simulink model "IEEE14_bus_system_2"  (R2024a)
settings: Solver=VariableStepAuto  StartTime=0.0  StopTime=0.2  RelTol=1e-3
libraries: spsThreePhaseSeriesRLCBranchLib x120, spsThreePhaseVIMeasurementLib x51, spsGroundLib x40, spsLoadFlowBusLib x33, spsThreePhaseSeriesRLCLoadLib x24, spsThreePhaseSourceLib x10, spsThreePhaseTransformerTwoWindingsLib x5, spspowerguiLib x2
(part 1 of 3)
settings Model: Creator=SIMPATY SOLUTIONS  LastModifiedBy=Nani
settings SolverCC: AlgebraicLoopSolver=TrustRegion
settings DebuggingCC: UnconnectedInputMsg=warning  UnconnectedOutputMsg=warning  UnconnectedLineMsg=warning
settings ModelReferenceCC: EnableRefExpFcnMdlSchedulingChecks=on
settings RTWCC: GPUComputeCapability=3.5

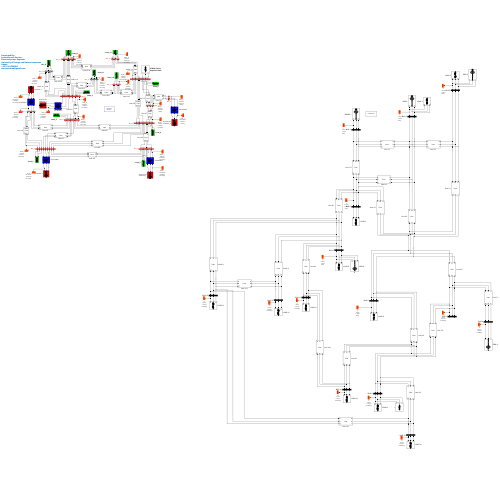
[thumbnail: Simulink's stored preview of the top-level diagram]
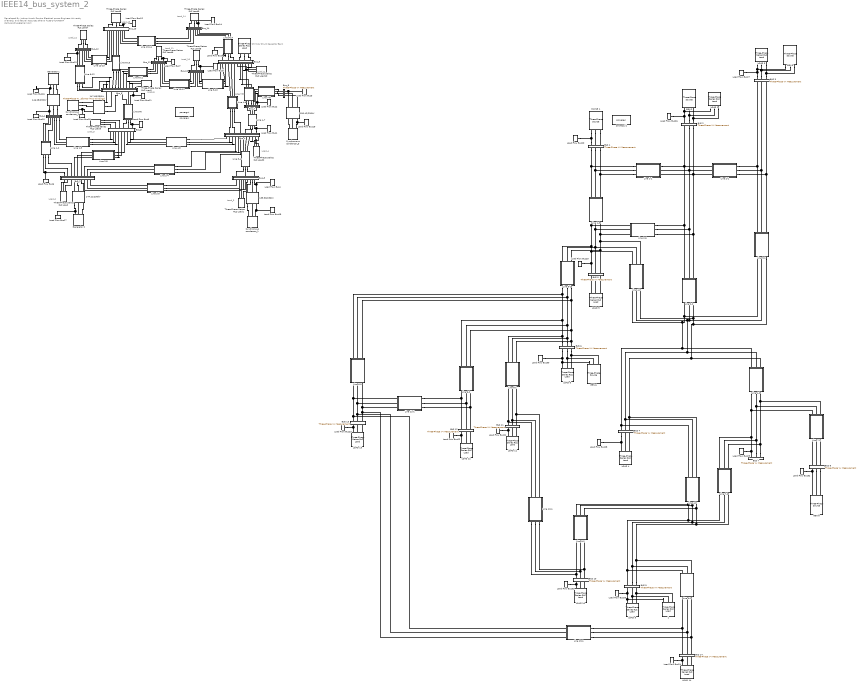
== system IEEE14_bus_system_2 ==
  note: Developed By:
      | Joshua Armah Dantuo
      | Electrical power Engineer
      | University of Energy and Natural resources
      | Ghana
      | +233-241790004
      | dantuojoshua@gmail.com
  note: 25 MVar Shunt
      | Capacitor Bank
  note: Load_4
  note: Load_3
  note: Load_5
  note: Load_9
  note: Load_11
  note: Load_10
  note: Load_12
  note: Load_6
  note: Load_13
  note: Load_14
  note: Load_2
  " " : spsThreePhaseSeriesRLCLoadLib/Three-Phase Series RLC Load  LConnTagsString=A|B|C  Configuration=Y (grounded)  NominalVoltage=230e3  Vabc=[1e3 1e3 1e3]  Vabcp=[1e3 1e3 1e3]  NominalFrequency=60  UnbalancedPower=off  ActivePower=0  InductivePower=0  CapacitivePower=25e6  Pabc=[10e3 9e3 11e3]  QLabc=[100 90 110]  QCabc=[100 90 110]  Pabcp=[10e3 9e3 11e3]  QLabcp=[100 90 110]  QCabcp=[100 90 110]  Measurements=None  LoadType=constant Z
  " 1" : spsThreePhaseSeriesRLCLoadLib/Three-Phase Series RLC Load  LConnTagsString=A|B|C  Configuration=Y (grounded)  NominalVoltage=230e3  Vabc=[1e3 1e3 1e3]  Vabcp=[1e3 1e3 1e3]  NominalFrequency=60  UnbalancedPower=off  ActivePower=0  InductivePower=0  CapacitivePower=25e6  Pabc=[10e3 9e3 11e3]  QLabc=[100 90 110]  QCabc=[100 90 110]  Pabcp=[10e3 9e3 11e3]  QLabcp=[100 90 110]  QCabcp=[100 90 110]  Measurements=None  LoadType=constant Z
  139.38/230kV : spsThreePhaseTransformerTwoWindingsLib/Three-Phase Transformer (Two Windings)  Winding1Connection=Yg  Winding2Connection=Yg  CoreType=Three single-phase transformers  SetSaturation=off  Hysteresis=off  DataFile='hysteresis'  SetInitialFlux=off  Measurements=None  UNITS=pu  NominalPower=[ 120e6 , 60 ]  Winding1=[139.38e3 , 0.002 , 0.08 ]  Winding2=[ 230e3 , 0.002 , 0.08 ]  Rm=500  Lm=500  L0=0.5  Saturation=[ 0,0 ; 0.0024,1.2 ; 1.0,1.52 ]  InitialFluxes=[ 0.8 , -0.8 , 0.7 ]  BreakLoop=off  DiscreteSolver=Trapezoidal iterative  DataType=off  TransfoNumber=1
  144.21/230kV : spsThreePhaseTransformerTwoWindingsLib/Three-Phase Transformer (Two Windings)  Winding1Connection=Yg  Winding2Connection=Yg  CoreType=Three single-phase transformers  SetSaturation=off  Hysteresis=off  DataFile='hysteresis'  SetInitialFlux=off  Measurements=None  UNITS=pu  NominalPower=[ 120e6 , 60 ]  Winding1=[144.21e3 , 0.002 , 0.08 ]  Winding2=[ 230e3 , 0.002 , 0.08 ]  Rm=500  Lm=500  L0=0.5  Saturation=[ 0,0 ; 0.0024,1.2 ; 1.0,1.52 ]  InitialFluxes=[ 0.8 , -0.8 , 0.7 ]  BreakLoop=off  DiscreteSolver=Trapezoidal iterative  DataType=off  TransfoNumber=1
  146.28/230kV : spsThreePhaseTransformerTwoWindingsLib/Three-Phase Transformer (Two Windings)  Winding1Connection=Yg  Winding2Connection=Yg  CoreType=Three single-phase transformers  SetSaturation=off  Hysteresis=off  DataFile='hysteresis'  SetInitialFlux=off  Measurements=None  UNITS=pu  NominalPower=[ 120e6 , 60 ]  Winding1=[146.28e3 , 0.002 , 0.08 ]  Winding2=[ 230e3 , 0.002 , 0.08 ]  Rm=500  Lm=500  L0=0.5  Saturation=[ 0,0 ; 0.0024,1.2 ; 1.0,1.52 ]  InitialFluxes=[ 0.8 , -0.8 , 0.7 ]  BreakLoop=off  DiscreteSolver=Trapezoidal iterative  DataType=off  TransfoNumber=1
  147.66/230kV : spsThreePhaseTransformerTwoWindingsLib/Three-Phase Transformer (Two Windings)  Winding1Connection=Yg  Winding2Connection=Yg  CoreType=Three single-phase transformers  SetSaturation=off  Hysteresis=off  DataFile='hysteresis'  SetInitialFlux=off  Measurements=None  UNITS=pu  NominalPower=[ 120e6 , 60 ]  Winding1=[147.66e3 , 0.002 , 0.08 ]  Winding2=[ 230e3 , 0.002 , 0.08 ]  Rm=500  Lm=500  L0=0.5  Saturation=[ 0,0 ; 0.0024,1.2 ; 1.0,1.52 ]  InitialFluxes=[ 0.8 , -0.8 , 0.7 ]  BreakLoop=off  DiscreteSolver=Trapezoidal iterative  DataType=off  TransfoNumber=1
  150.42/230kV : spsThreePhaseTransformerTwoWindingsLib/Three-Phase Transformer (Two Windings)  Winding1Connection=Yg  Winding2Connection=Yg  CoreType=Three single-phase transformers  SetSaturation=off  Hysteresis=off  DataFile='hysteresis'  SetInitialFlux=off  Measurements=None  UNITS=pu  NominalPower=[ 120e6 , 60 ]  Winding1=[150.42e3 , 0.002 , 0.08 ]  Winding2=[ 230e3 , 0.002 , 0.08 ]  Rm=500  Lm=500  L0=0.5  Saturation=[ 0,0 ; 0.0024,1.2 ; 1.0,1.52 ]  InitialFluxes=[ 0.8 , -0.8 , 0.7 ]  BreakLoop=off  DiscreteSolver=Trapezoidal iterative  DataType=off  TransfoNumber=1
  BUS {1..14} (14 alike) : spsThreePhaseVIMeasurementLib/Three-Phase V-I Measurement  VoltageMeasurement=no  SetLabelV=off  LabelV=Vabc  Vpu=off  VpuLL=off  CurrentMeasurement=no  SetLabelI=off  LabelI=Iabc  Ipu=off  Pbase=100e6  Vbase=500e3  OutputType=Complex  PhasorSimulation=off  PSBequivalent=0
  Bus_1 : Subsystem
  Bus_10 : Subsystem
  Bus_11 : Subsystem
  Bus_12 : Subsystem
  Bus_13 : Subsystem
  Bus_14 : Subsystem
  Bus_2 : Subsystem
  Bus_3 : Subsystem
  Bus_4 : Subsystem
  Bus_5 : Subsystem
  Bus_6 : Subsystem
  Bus_7 : Subsystem
  Bus_8 : spsThreePhaseVIMeasurementLib/Three-Phase V-I Measurement  VoltageMeasurement=phase-to-phase  SetLabelV=on  LabelV=VB_8  Vpu=off  VpuLL=off  CurrentMeasurement=yes  SetLabelI=on  LabelI=IB_8  Ipu=off  Pbase=100e6  Vbase=500e3  OutputType=Complex  PhasorSimulation=off  PSBequivalent=0
  Bus_9 : Subsystem
  GEN 2 : spsThreePhaseSourceLib/Three-Phase Source  InternalConnection=Yg  VoltagePhases=off  Voltage=(10000)*1.045  PhaseAngle=0  Voltage_phases=[25e3 25e3 25e3]/sqrt(3)  PhaseAngles_phases=[0 -120 +120]  Frequency=60  NonIdealSource=off  SpecifyImpedance=off  Resistance=0.8929  Inductance=16.58e-3  ShortCircuitLevel=100e6  BaseVoltage=25e3  XRratio=7  BusType=PV  Pref=40e6  Qref=0  Prefabc=[10e3, 10e3, 10e3]  Qrefabc=[0, 0, 0]  Qmin=-40e6  Qmax=50e6
  GEN 3 : spsThreePhaseSourceLib/Three-Phase Source  InternalConnection=Yg  VoltagePhases=off  Voltage=(10000)*1.01  PhaseAngle=0  Voltage_phases=[25e3 25e3 25e3]/sqrt(3)  PhaseAngles_phases=[0 -120 +120]  Frequency=60  NonIdealSource=off  SpecifyImpedance=off  Resistance=0.8929  Inductance=16.58e-3  ShortCircuitLevel=100e6  BaseVoltage=25e3  XRratio=7  BusType=PV  Pref=0  Qref=0  Prefabc=[10e3, 10e3, 10e3]  Qrefabc=[0, 0, 0]  Qmin=0  Qmax=40e6
  GEN 6 : spsThreePhaseSourceLib/Three-Phase Source  InternalConnection=Yn  VoltagePhases=off  Voltage=(10000)*1.070  PhaseAngle=0  Voltage_phases=[25e3 25e3 25e3]/sqrt(3)  PhaseAngles_phases=[0 -120 +120]  Frequency=60  NonIdealSource=off  SpecifyImpedance=off  Resistance=0.8929  Inductance=16.58e-3  ShortCircuitLevel=100e6  BaseVoltage=25e3  XRratio=7  BusType=PV  Pref=0  Qref=7.5e6  Prefabc=[10e3, 10e3, 10e3]  Qrefabc=[0, 0, 0]  Qmin=-6e6  Qmax=24e6
  GEN 8 : spsThreePhaseSourceLib/Three-Phase Source  InternalConnection=Yn  VoltagePhases=off  Voltage=(10000)*1.090  PhaseAngle=0  Voltage_phases=[25e3 25e3 25e3]/sqrt(3)  PhaseAngles_phases=[0 -120 +120]  Frequency=60  NonIdealSource=off  SpecifyImpedance=off  Resistance=0.8929  Inductance=16.58e-3  ShortCircuitLevel=100e6  BaseVoltage=25e3  XRratio=7  BusType=PV  Pref=0  Qref=30e6  Prefabc=[10e3, 10e3, 10e3]  Qrefabc=[0, 0, 0]  Qmin=-6e6  Qmax=24e6
  Generator 1 : spsThreePhaseSourceLib/Three-Phase Source  InternalConnection=Yg  VoltagePhases=off  Voltage=(146280)*1.03071  PhaseAngle=3.7708  Voltage_phases=[25e3 25e3 25e3]/sqrt(3)  PhaseAngles_phases=[0 -120 +120]  Frequency=60  NonIdealSource=on  SpecifyImpedance=off  Resistance=0.8929  Inductance=16.58e-3  ShortCircuitLevel=100e6  BaseVoltage=146.28e3  XRratio=7  BusType=swing  Pref=163e6  Qref=0  Prefabc=[10e3, 10e3, 10e3]  Qrefabc=[0, 0, 0]  Qmin=-inf  Qmax=inf
  Generator 2 : spsThreePhaseSourceLib/Three-Phase Source  InternalConnection=Yg  VoltagePhases=off  Voltage=(144210)*1.045  PhaseAngle=-15.8323  Voltage_phases=[25e3 25e3 25e3]/sqrt(3)  PhaseAngles_phases=[0 -120 +120]  Frequency=60  NonIdealSource=on  SpecifyImpedance=off  Resistance=0.8929  Inductance=16.58e-3  ShortCircuitLevel=100e6  BaseVoltage=144.21e3  XRratio=7  BusType=PV  Pref=90e6  Qref=0  Prefabc=[10e3, 10e3, 10e3]  Qrefabc=[0, 0, 0]  Qmin=-40e6  Qmax=50e6
  LOAD 10 : spsThreePhaseSeriesRLCLoadLib/Three-Phase Series RLC Load  LConnTagsString=A|B|C  Configuration=Y (grounded)  NominalVoltage=(10000)*1.01794  Vabc=[1e3 1e3 1e3]  Vabcp=[1e3 1e3 1e3]  NominalFrequency=60  UnbalancedPower=off  ActivePower=9e6  InductivePower=5.8e6  CapacitivePower=0  Pabc=[10e3 9e3 11e3]  QLabc=[100 90 110]  QCabc=[100 90 110]  Pabcp=[10e3 9e3 11e3]  QLabcp=[100 90 110]  QCabcp=[100 90 110]  Measurements=None  LoadType=constant PQ
  LOAD 11 : spsThreePhaseSeriesRLCLoadLib/Three-Phase Series RLC Load  LConnTagsString=A|B|C  Configuration=Y (grounded)  NominalVoltage=(10000)*1.01794  Vabc=[1e3 1e3 1e3]  Vabcp=[1e3 1e3 1e3]  NominalFrequency=60  UnbalancedPower=off  ActivePower=3.5e6  InductivePower=1.8e6  CapacitivePower=0  Pabc=[10e3 9e3 11e3]  QLabc=[100 90 110]  QCabc=[100 90 110]  Pabcp=[10e3 9e3 11e3]  QLabcp=[100 90 110]  QCabcp=[100 90 110]  Measurements=None  LoadType=constant PQ
  LOAD 12 : spsThreePhaseSeriesRLCLoadLib/Three-Phase Series RLC Load  LConnTagsString=A|B|C  Configuration=Y (grounded)  NominalVoltage=(10000)*1.01794  Vabc=[1e3 1e3 1e3]  Vabcp=[1e3 1e3 1e3]  NominalFrequency=60  UnbalancedPower=off  ActivePower=6.1e6  InductivePower=1.6e6  CapacitivePower=0  Pabc=[10e3 9e3 11e3]  QLabc=[100 90 110]  QCabc=[100 90 110]  Pabcp=[10e3 9e3 11e3]  QLabcp=[100 90 110]  QCabcp=[100 90 110]  Measurements=None  LoadType=constant PQ
  LOAD 13 : spsThreePhaseSeriesRLCLoadLib/Three-Phase Series RLC Load  LConnTagsString=A|B|C  Configuration=Y (grounded)  NominalVoltage=(10000)*1.01794  Vabc=[1e3 1e3 1e3]  Vabcp=[1e3 1e3 1e3]  NominalFrequency=60  UnbalancedPower=off  ActivePower=13.5e6  InductivePower=5.8e6  CapacitivePower=0  Pabc=[10e3 9e3 11e3]  QLabc=[100 90 110]  QCabc=[100 90 110]  Pabcp=[10e3 9e3 11e3]  QLabcp=[100 90 110]  QCabcp=[100 90 110]  Measurements=None  LoadType=constant PQ
  LOAD 14 : spsThreePhaseSeriesRLCLoadLib/Three-Phase Series RLC Load  LConnTagsString=A|B|C  Configuration=Y (grounded)  NominalVoltage=(10000)*1.01794  Vabc=[1e3 1e3 1e3]  Vabcp=[1e3 1e3 1e3]  NominalFrequency=60  UnbalancedPower=off  ActivePower=14.9e6  InductivePower=5e6  CapacitivePower=0  Pabc=[10e3 9e3 11e3]  QLabc=[100 90 110]  QCabc=[100 90 110]  Pabcp=[10e3 9e3 11e3]  QLabcp=[100 90 110]  QCabcp=[100 90 110]  Measurements=None  LoadType=constant PQ
  LOAD 2 : spsThreePhaseSeriesRLCLoadLib/Three-Phase Series RLC Load  LConnTagsString=A|B|C  Configuration=Y (grounded)  NominalVoltage=(10000)*1.01794  Vabc=[1e3 1e3 1e3]  Vabcp=[1e3 1e3 1e3]  NominalFrequency=60  UnbalancedPower=off  ActivePower=21.7e6  InductivePower=12.7e6  CapacitivePower=0  Pabc=[10e3 9e3 11e3]  QLabc=[100 90 110]  QCabc=[100 90 110]  Pabcp=[10e3 9e3 11e3]  QLabcp=[100 90 110]  QCabcp=[100 90 110]  Measurements=None  LoadType=constant PQ
  LOAD 3 : spsThreePhaseSeriesRLCLoadLib/Three-Phase Series RLC Load  LConnTagsString=A|B|C  Configuration=Y (grounded)  NominalVoltage=(10000)*1.01794  Vabc=[1e3 1e3 1e3]  Vabcp=[1e3 1e3 1e3]  NominalFrequency=60  UnbalancedPower=off  ActivePower=94.2e6  InductivePower=19e6  CapacitivePower=0  Pabc=[10e3 9e3 11e3]  QLabc=[100 90 110]  QCabc=[100 90 110]  Pabcp=[10e3 9e3 11e3]  QLabcp=[100 90 110]  QCabcp=[100 90 110]  Measurements=None  LoadType=constant PQ
  LOAD 4 : spsThreePhaseSeriesRLCLoadLib/Three-Phase Series RLC Load  LConnTagsString=A|B|C  Configuration=Y (grounded)  NominalVoltage=(10000)*1.01794  Vabc=[1e3 1e3 1e3]  Vabcp=[1e3 1e3 1e3]  NominalFrequency=60  UnbalancedPower=off  ActivePower=47.8e6  InductivePower=0  CapacitivePower=3.9e6  Pabc=[10e3 9e3 11e3]  QLabc=[100 90 110]  QCabc=[100 90 110]  Pabcp=[10e3 9e3 11e3]  QLabcp=[100 90 110]  QCabcp=[100 90 110]  Measurements=None  LoadType=constant PQ
  LOAD 5 : spsThreePhaseSeriesRLCLoadLib/Three-Phase Series RLC Load  LConnTagsString=A|B|C  Configuration=Y (grounded)  NominalVoltage=(10000)*1.01794  Vabc=[1e3 1e3 1e3]  Vabcp=[1e3 1e3 1e3]  NominalFrequency=60  UnbalancedPower=off  ActivePower=7.6e6  InductivePower=1.6e6  CapacitivePower=0  Pabc=[10e3 9e3 11e3]  QLabc=[100 90 110]  QCabc=[100 90 110]  Pabcp=[10e3 9e3 11e3]  QLabcp=[100 90 110]  QCabcp=[100 90 110]  Measurements=None  LoadType=constant PQ
  LOAD 6 : spsThreePhaseSeriesRLCLoadLib/Three-Phase Series RLC Load  LConnTagsString=A|B|C  Configuration=Y (grounded)  NominalVoltage=(10000)*1.01794  Vabc=[1e3 1e3 1e3]  Vabcp=[1e3 1e3 1e3]  NominalFrequency=60  UnbalancedPower=off  ActivePower=11.2e6  InductivePower=7.5e6  CapacitivePower=0  Pabc=[10e3 9e3 11e3]  QLabc=[100 90 110]  QCabc=[100 90 110]  Pabcp=[10e3 9e3 11e3]  QLabcp=[100 90 110]  QCabcp=[100 90 110]  Measurements=None  LoadType=constant PQ
  LOAD 9 : spsThreePhaseSeriesRLCLoadLib/Three-Phase Series RLC Load  LConnTagsString=A|B|C  Configuration=Y (grounded)  NominalVoltage=(10000)*1.01794  Vabc=[1e3 1e3 1e3]  Vabcp=[1e3 1e3 1e3]  NominalFrequency=60  UnbalancedPower=off  ActivePower=29.5e6  InductivePower=16.6e6  CapacitivePower=0  Pabc=[10e3 9e3 11e3]  QLabc=[100 90 110]  QCabc=[100 90 110]  Pabcp=[10e3 9e3 11e3]  QLabcp=[100 90 110]  QCabcp=[100 90 110]  Measurements=None  LoadType=constant PQ
  Line 1-1 : Subsystem  mask{F=60, R=0.01938, xL=0.05917, B=0.02640}
      mask prompts: F "Line Frequency (Hz)"; R "Line Resistance (pu)"; xL "Line Inductance (pu)"; B "Line Susceptance (pu)"
      mask Display:
      | disp('Line');
      | port_label('lconn',1,'A');
      | port_label('lconn',2,'B');
      | port_label('lconn',3,'C');
      | port_label('rconn',1,'a');
      | port_label('rconn',2,'b');
      | port_label('rconn',3,'c');
  Line 1-2 : Subsystem  mask{F=60, R=0.04699, xL=0.19797, B=0.02190}
      mask prompts: F "Line Frequency (Hz)"; R "Line Resistance (pu)"; xL "Line Inductance (pu)"; B "Line Susceptance (pu)"
      mask Display:
      | disp('Line');
      | port_label('lconn',1,'A');
      | port_label('lconn',2,'B');
      | port_label('lconn',3,'C');
      | port_label('rconn',1,'a');
      | port_label('rconn',2,'b');
      | port_label('rconn',3,'c');
  Line 1-3 : Subsystem  mask{F=60, R=0.05403, xL=0.22304, B=0.02460}
      mask prompts: F "Line Frequency (Hz)"; R "Line Resistance (pu)"; xL "Line Inductance (pu)"; B "Line Susceptance (pu)"
      mask Display:
      | disp('Line');
      | port_label('lconn',1,'A');
      | port_label('lconn',2,'B');
      | port_label('lconn',3,'C');
      | port_label('rconn',1,'a');
      | port_label('rconn',2,'b');
      | port_label('rconn',3,'c');
  Line 1-5 : Subsystem  mask{F=60, R=0.05403, xL=0.22304, B=0.02460}
      mask prompts: F "Line Frequency (Hz)"; R "Line Resistance (pu)"; xL "Line Inductance (pu)"; B "Line Susceptance (pu)"
      mask Display:
      | disp('Line');
      | port_label('lconn',1,'A');
      | port_label('lconn',2,'B');
      | port_label('lconn',3,'C');
      | port_label('rconn',1,'a');
      | port_label('rconn',2,'b');
      | port_label('rconn',3,'c');
  Line 10-1 : Subsystem  mask{F=60, R=0.08205, xL=0.19207, B=0}
      mask prompts: F "Line Frequency (Hz)"; R "Line Resistance (pu)"; xL "Line Inductance (pu)"; B "Line Susceptance (pu)"
      mask Display:
      | disp('Line');
      | port_label('lconn',1,'A');
      | port_label('lconn',2,'B');
      | port_label('lconn',3,'C');
      | port_label('rconn',1,'a');
      | port_label('rconn',2,'b');
      | port_label('rconn',3,'c');
  Line 10-11 : Subsystem  mask{F=60, R=0.08205, xL=0.19207, B=0}
      mask prompts: F "Line Frequency (Hz)"; R "Line Resistance (pu)"; xL "Line Inductance (pu)"; B "Line Susceptance (pu)"
      mask Display:
      | disp('Line');
      | port_label('lconn',1,'A');
      | port_label('lconn',2,'B');
      | port_label('lconn',3,'C');
      | port_label('rconn',1,'a');
      | port_label('rconn',2,'b');
      | port_label('rconn',3,'c');
  Line 12-1 : Subsystem  mask{F=60, R=0.22092, xL=0.19988, B=0}
      mask prompts: F "Line Frequency (Hz)"; R "Line Resistance (pu)"; xL "Line Inductance (pu)"; B "Line Susceptance (pu)"
      mask Display:
      | disp('Line');
      | port_label('lconn',1,'A');
      | port_label('lconn',2,'B');
      | port_label('lconn',3,'C');
      | port_label('rconn',1,'a');
      | port_label('rconn',2,'b');
      | port_label('rconn',3,'c');
  Line 12-13 : Subsystem  mask{F=60, R=0.22092, xL=0.19988, B=0}
      mask prompts: F "Line Frequency (Hz)"; R "Line Resistance (pu)"; xL "Line Inductance (pu)"; B "Line Susceptance (pu)"
      mask Display:
      | disp('Line');
      | port_label('lconn',1,'A');
      | port_label('lconn',2,'B');
      | port_label('lconn',3,'C');
      | port_label('rconn',1,'a');
      | port_label('rconn',2,'b');
      | port_label('rconn',3,'c');
  Line 13-1 : Subsystem  mask{F=60, R=0.17093, xL=0.34802, B=0}
      mask prompts: F "Line Frequency (Hz)"; R "Line Resistance (pu)"; xL "Line Inductance (pu)"; B "Line Susceptance (pu)"
      mask Display:
      | disp('Line');
      | port_label('lconn',1,'A');
      | port_label('lconn',2,'B');
      | port_label('lconn',3,'C');
      | port_label('rconn',1,'a');
      | port_label('rconn',2,'b');
      | port_label('rconn',3,'c');
  Line 13-14 : Subsystem  mask{F=60, R=0.17093, xL=0.34802, B=0}
      mask prompts: F "Line Frequency (Hz)"; R "Line Resistance (pu)"; xL "Line Inductance (pu)"; B "Line Susceptance (pu)"
      mask Display:
      | disp('Line');
      | port_label('lconn',1,'A');
      | port_label('lconn',2,'B');
      | port_label('lconn',3,'C');
      | port_label('rconn',1,'a');
      | port_label('rconn',2,'b');
      | port_label('rconn',3,'c');
  Line 2-1 : Subsystem  mask{F=60, R=0.04699, xL=0.19797, B=0.02190}
      mask prompts: F "Line Frequency (Hz)"; R "Line Resistance (pu)"; xL "Line Inductance (pu)"; B "Line Susceptance (pu)"
      mask Display:
      | disp('Line');
      | port_label('lconn',1,'A');
      | port_label('lconn',2,'B');
      | port_label('lconn',3,'C');
      | port_label('rconn',1,'a');
      | port_label('rconn',2,'b');
      | port_label('rconn',3,'c');
  Line 2-2 : Subsystem  mask{F=60, R=0.05811, xL=0.17632, B=0.01870}
      mask prompts: F "Line Frequency (Hz)"; R "Line Resistance (pu)"; xL "Line Inductance (pu)"; B "Line Susceptance (pu)"
      mask Display:
      | disp('Line');
      | port_label('lconn',1,'A');
      | port_label('lconn',2,'B');
      | port_label('lconn',3,'C');
      | port_label('rconn',1,'a');
      | port_label('rconn',2,'b');
      | port_label('rconn',3,'c');
  Line 2-3 : Subsystem  mask{F=60, R=0.04699, xL=0.19797, B=0.02190}
      mask prompts: F "Line Frequency (Hz)"; R "Line Resistance (pu)"; xL "Line Inductance (pu)"; B "Line Susceptance (pu)"
      mask Display:
      | disp('Line');
      | port_label('lconn',1,'A');
      | port_label('lconn',2,'B');
      | port_label('lconn',3,'C');
      | port_label('rconn',1,'a');
      | port_label('rconn',2,'b');
      | port_label('rconn',3,'c');
  Line 2-4 : Subsystem  mask{F=60, R=0.05811, xL=0.17632, B=0.01870}
      mask prompts: F "Line Frequency (Hz)"; R "Line Resistance (pu)"; xL "Line Inductance (pu)"; B "Line Susceptance (pu)"
      mask Display:
      | disp('Line');
      | port_label('lconn',1,'A');
      | port_label('lconn',2,'B');
      | port_label('lconn',3,'C');
      | port_label('rconn',1,'a');
      | port_label('rconn',2,'b');
      | port_label('rconn',3,'c');
  Line 2-5 : Subsystem  mask{F=60, R=0.05695, xL=0.17388, B=0.01700}
      mask prompts: F "Line Frequency (Hz)"; R "Line Resistance (pu)"; xL "Line Inductance (pu)"; B "Line Susceptance (pu)"
      mask Display:
      | disp('Line');
      | port_label('lconn',1,'A');
      | port_label('lconn',2,'B');
      | port_label('lconn',3,'C');
      | port_label('rconn',1,'a');
      | port_label('rconn',2,'b');
      | port_label('rconn',3,'c');
  Line 2-6 : Subsystem  mask{F=60, R=0.05695, xL=0.17388, B=0.01700}
      mask prompts: F "Line Frequency (Hz)"; R "Line Resistance (pu)"; xL "Line Inductance (pu)"; B "Line Susceptance (pu)"
      mask Display:
      | disp('Line');
      | port_label('lconn',1,'A');
      | port_label('lconn',2,'B');
      | port_label('lconn',3,'C');
      | port_label('rconn',1,'a');
      | port_label('rconn',2,'b');
      | port_label('rconn',3,'c');
  Line 3-1 : Subsystem  mask{F=60, R=0.06701, xL=0.17103, B=0.01730}
      mask prompts: F "Line Frequency (Hz)"; R "Line Resistance (pu)"; xL "Line Inductance (pu)"; B "Line Susceptance (pu)"
      mask Display:
      | disp('Line');
      | port_label('lconn',1,'A');
      | port_label('lconn',2,'B');
      | port_label('lconn',3,'C');
      | port_label('rconn',1,'a');
      | port_label('rconn',2,'b');
      | port_label('rconn',3,'c');
  Line 3-4 : Subsystem  mask{F=60, R=0.06701, xL=0.17103, B=0.01730}
      mask prompts: F "Line Frequency (Hz)"; R "Line Resistance (pu)"; xL "Line Inductance (pu)"; B "Line Susceptance (pu)"
      mask Display:
      | disp('Line');
      | port_label('lconn',1,'A');
      | port_label('lconn',2,'B');
      | port_label('lconn',3,'C');
      | port_label('rconn',1,'a');
      | port_label('rconn',2,'b');
      | port_label('rconn',3,'c');
  Line 4-1 : Subsystem  mask{F=60, R=0.01335, xL=0.04211, B=0.0064}
      mask prompts: F "Line Frequency (Hz)"; R "Line Resistance (pu)"; xL "Line Inductance (pu)"; B "Line Susceptance (pu)"
      mask Display:
      | disp('Line');
      | port_label('lconn',1,'A');
      | port_label('lconn',2,'B');
      | port_label('lconn',3,'C');
      | port_label('rconn',1,'a');
      | port_label('rconn',2,'b');
      | port_label('rconn',3,'c');
  Line 4-2 : Subsystem  mask{F=60, R=0, xL=0.20912, B=0}
      mask prompts: F "Line Frequency (Hz)"; R "Line Resistance (pu)"; xL "Line Inductance (pu)"; B "Line Susceptance (pu)"
      mask Display:
      | disp('Line');
      | port_label('lconn',1,'A');
      | port_label('lconn',2,'B');
      | port_label('lconn',3,'C');
      | port_label('rconn',1,'a');
      | port_label('rconn',2,'b');
      | port_label('rconn',3,'c');
  Line 4-3 : Subsystem  mask{F=60, R=0, xL=0.55618, B=0}
      mask prompts: F "Line Frequency (Hz)"; R "Line Resistance (pu)"; xL "Line Inductance (pu)"; B "Line Susceptance (pu)"
      mask Display:
      | disp('Line');
      | port_label('lconn',1,'A');
      | port_label('lconn',2,'B');
      | port_label('lconn',3,'C');
      | port_label('rconn',1,'a');
      | port_label('rconn',2,'b');
      | port_label('rconn',3,'c');
  Line 4-5 : Subsystem  mask{F=60, R=0.01335, xL=0.04211, B=0.0064}
      mask prompts: F "Line Frequency (Hz)"; R "Line Resistance (pu)"; xL "Line Inductance (pu)"; B "Line Susceptance (pu)"
      mask Display:
      | disp('Line');
      | port_label('lconn',1,'A');
      | port_label('lconn',2,'B');
      | port_label('lconn',3,'C');
      | port_label('rconn',1,'a');
      | port_label('rconn',2,'b');
      | port_label('rconn',3,'c');
  Line 4-7 : Subsystem  mask{F=60, R=0, xL=0.20912, B=0}
      mask prompts: F "Line Frequency (Hz)"; R "Line Resistance (pu)"; xL "Line Inductance (pu)"; B "Line Susceptance (pu)"
      mask Display:
      | disp('Line');
      | port_label('lconn',1,'A');
      | port_label('lconn',2,'B');
      | port_label('lconn',3,'C');
      | port_label('rconn',1,'a');
      | port_label('rconn',2,'b');
      | port_label('rconn',3,'c');
  Line 4-9 : Subsystem  mask{F=60, R=0, xL=0.55618, B=0}
      mask prompts: F "Line Frequency (Hz)"; R "Line Resistance (pu)"; xL "Line Inductance (pu)"; B "Line Susceptance (pu)"
      mask Display:
      | disp('Line');
      | port_label('lconn',1,'A');
      | port_label('lconn',2,'B');
      | port_label('lconn',3,'C');
      | port_label('rconn',1,'a');
      | port_label('rconn',2,'b');
      | port_label('rconn',3,'c');
  Line 5-1 : Subsystem  mask{F=60, R=0, xL=0.25202, B=0}
      mask prompts: F "Line Frequency (Hz)"; R "Line Resistance (pu)"; xL "Line Inductance (pu)"; B "Line Susceptance (pu)"
      mask Display:
      | disp('Line');
      | port_label('lconn',1,'A');
      | port_label('lconn',2,'B');
      | port_label('lconn',3,'C');
      | port_label('rconn',1,'a');
      | port_label('rconn',2,'b');
      | port_label('rconn',3,'c');
  Line 5-6 : Subsystem  mask{F=60, R=0, xL=0.25202, B=0}
      mask prompts: F "Line Frequency (Hz)"; R "Line Resistance (pu)"; xL "Line Inductance (pu)"; B "Line Susceptance (pu)"
      mask Display:
      | disp('Line');
      | port_label('lconn',1,'A');
      | port_label('lconn',2,'B');
      | port_label('lconn',3,'C');
      | port_label('rconn',1,'a');
      | port_label('rconn',2,'b');
      | port_label('rconn',3,'c');
  Line 6-1 : Subsystem  mask{F=60, R=0.09498, xL=0.19890, B=0}
      mask prompts: F "Line Frequency (Hz)"; R "Line Resistance (pu)"; xL "Line Inductance (pu)"; B "Line Susceptance (pu)"
      mask Display:
      | disp('Line');
      | port_label('lconn',1,'A');
      | port_label('lconn',2,'B');
      | port_label('lconn',3,'C');
      | port_label('rconn',1,'a');
      | port_label('rconn',2,'b');
      | port_label('rconn',3,'c');
  Line 6-11 : Subsystem  mask{F=60, R=0.09498, xL=0.19890, B=0}
      mask prompts: F "Line Frequency (Hz)"; R "Line Resistance (pu)"; xL "Line Inductance (pu)"; B "Line Susceptance (pu)"
      mask Display:
      | disp('Line');
      | port_label('lconn',1,'A');
      | port_label('lconn',2,'B');
      | port_label('lconn',3,'C');
      | port_label('rconn',1,'a');
      | port_label('rconn',2,'b');
      | port_label('rconn',3,'c');
  Line 6-12 : Subsystem  mask{F=60, R=0.12291, xL=0.25581, B=0}
      mask prompts: F "Line Frequency (Hz)"; R "Line Resistance (pu)"; xL "Line Inductance (pu)"; B "Line Susceptance (pu)"
      mask Display:
      | disp('Line');
      | port_label('lconn',1,'A');
      | port_label('lconn',2,'B');
      | port_label('lconn',3,'C');
      | port_label('rconn',1,'a');
      | port_label('rconn',2,'b');
      | port_label('rconn',3,'c');
  Line 6-13 : Subsystem  mask{F=60, R=0.06615, xL=0.13027, B=0}
      mask prompts: F "Line Frequency (Hz)"; R "Line Resistance (pu)"; xL "Line Inductance (pu)"; B "Line Susceptance (pu)"
      mask Display:
      | disp('Line');
      | port_label('lconn',1,'A');
      | port_label('lconn',2,'B');
      | port_label('lconn',3,'C');
      | port_label('rconn',1,'a');
      | port_label('rconn',2,'b');
      | port_label('rconn',3,'c');
  Line 6-2 : Subsystem  mask{F=60, R=0.12291, xL=0.25581, B=0}
      mask prompts: F "Line Frequency (Hz)"; R "Line Resistance (pu)"; xL "Line Inductance (pu)"; B "Line Susceptance (pu)"
      mask Display:
      | disp('Line');
      | port_label('lconn',1,'A');
      | port_label('lconn',2,'B');
      | port_label('lconn',3,'C');
      | port_label('rconn',1,'a');
      | port_label('rconn',2,'b');
      | port_label('rconn',3,'c');
  Line 6-3 : Subsystem  mask{F=60, R=0.06615, xL=0.13027, B=0}
      mask prompts: F "Line Frequency (Hz)"; R "Line Resistance (pu)"; xL "Line Inductance (pu)"; B "Line Susceptance (pu)"
      mask Display:
      | disp('Line');
      | port_label('lconn',1,'A');
      | port_label('lconn',2,'B');
      | port_label('lconn',3,'C');
      | port_label('rconn',1,'a');
      | port_label('rconn',2,'b');
      | port_label('rconn',3,'c');
  Line 7-1 : Subsystem  mask{F=60, R=0, xL=0.17615, B=0}
      mask prompts: F "Line Frequency (Hz)"; R "Line Resistance (pu)"; xL "Line Inductance (pu)"; B "Line Susceptance (pu)"
      mask Display:
      | disp('Line');
      | port_label('lconn',1,'A');
      | port_label('lconn',2,'B');
      | port_label('lconn',3,'C');
      | port_label('rconn',1,'a');
      | port_label('rconn',2,'b');
      | port_label('rconn',3,'c');
  Line 7-2 : Subsystem  mask{F=60, R=0, xL=0.11001, B=0}
      mask prompts: F "Line Frequency (Hz)"; R "Line Resistance (pu)"; xL "Line Inductance (pu)"; B "Line Susceptance (pu)"
      mask Display:
      | disp('Line');
      | port_label('lconn',1,'A');
      | port_label('lconn',2,'B');
      | port_label('lconn',3,'C');
      | port_label('rconn',1,'a');
      | port_label('rconn',2,'b');
      | port_label('rconn',3,'c');
  Line 7-8 : Subsystem  mask{F=60, R=0, xL=0.17615, B=0}
      mask prompts: F "Line Frequency (Hz)"; R "Line Resistance (pu)"; xL "Line Inductance (pu)"; B "Line Susceptance (pu)"
      mask Display:
      | disp('Line');
      | port_label('lconn',1,'A');
      | port_label('lconn',2,'B');
      | port_label('lconn',3,'C');
      | port_label('rconn',1,'a');
      | port_label('rconn',2,'b');
      | port_label('rconn',3,'c');
  Line 7-9 : Subsystem  mask{F=60, R=0, xL=0.11001, B=0}
      mask prompts: F "Line Frequency (Hz)"; R "Line Resistance (pu)"; xL "Line Inductance (pu)"; B "Line Susceptance (pu)"
      mask Display:
      | disp('Line');
      | port_label('lconn',1,'A');
      | port_label('lconn',2,'B');
      | port_label('lconn',3,'C');
      | port_label('rconn',1,'a');
      | port_label('rconn',2,'b');
      | port_label('rconn',3,'c');
  Line 9-1 : Subsystem  mask{F=60, R=0.03181, xL=0.08450, B=0}
      mask prompts: F "Line Frequency (Hz)"; R "Line Resistance (pu)"; xL "Line Inductance (pu)"; B "Line Susceptance (pu)"
      mask Display:
      | disp('Line');
      | port_label('lconn',1,'A');
      | port_label('lconn',2,'B');
      | port_label('lconn',3,'C');
      | port_label('rconn',1,'a');
      | port_label('rconn',2,'b');
      | port_label('rconn',3,'c');
  Line 9-10 : Subsystem  mask{F=60, R=0.03181, xL=0.08450, B=0}
      mask prompts: F "Line Frequency (Hz)"; R "Line Resistance (pu)"; xL "Line Inductance (pu)"; B "Line Susceptance (pu)"
      mask Display:
      | disp('Line');
      | port_label('lconn',1,'A');
      | port_label('lconn',2,'B');
      | port_label('lconn',3,'C');
      | port_label('rconn',1,'a');
      | port_label('rconn',2,'b');
      | port_label('rconn',3,'c');
  Line 9-14 : Subsystem  mask{F=60, R=0.12711, xL=0.27038, B=0}
      mask prompts: F "Line Frequency (Hz)"; R "Line Resistance (pu)"; xL "Line Inductance (pu)"; B "Line Susceptance (pu)"
      mask Display:
      | disp('Line');
      | port_label('lconn',1,'A');
      | port_label('lconn',2,'B');
      | port_label('lconn',3,'C');
      | port_label('rconn',1,'a');
      | port_label('rconn',2,'b');
      | port_label('rconn',3,'c');
  Line 9-2 : Subsystem  mask{F=60, R=0.12711, xL=0.27038, B=0}
      mask prompts: F "Line Frequency (Hz)"; R "Line Resistance (pu)"; xL "Line Inductance (pu)"; B "Line Susceptance (pu)"
      mask Display:
      | disp('Line');
      | port_label('lconn',1,'A');
      | port_label('lconn',2,'B');
      | port_label('lconn',3,'C');
      | port_label('rconn',1,'a');
      | port_label('rconn',2,'b');
      | port_label('rconn',3,'c');
  Load Flow Bus1 : spsLoadFlowBusLib/Load Flow Bus  LConnTagsString=a  Phases=single  Connectors=on one side  ID=BUS_4  Vbase=230e3  Vref=1.019  Vangle=0  VLF=0.928  VLFb=1  VLFc=1  angleLF=-31.28  angleLFb=0  angleLFc=0
  Load Flow Bus10 : spsLoadFlowBusLib/Load Flow Bus  LConnTagsString=a  Phases=single  Connectors=on one side  ID=BUS_1  Vbase=230e3  Vref=1.060  Vangle=0  VLF=0.9625  VLFb=1  VLFc=1  angleLF=-19.37  angleLFb=0  angleLFc=0
  Load Flow Bus11 : spsLoadFlowBusLib/Load Flow Bus  LConnTagsString=a  Phases=single  Connectors=on one side  ID=BUS_6  Vbase=230e3  Vref=1.070  Vangle=0  VLF=0.9425  VLFb=1  VLFc=1  angleLF=-36.08  angleLFb=0  angleLFc=0
  Load Flow Bus12 : spsLoadFlowBusLib/Load Flow Bus  LConnTagsString=a  Phases=single  Connectors=on one side  ID=BUS_13  Vbase=230e3  Vref=1.050  Vangle=0  VLF=0.9416  VLFb=1  VLFc=1  angleLF=-36.14  angleLFb=0  angleLFc=0
  Load Flow Bus13 : spsLoadFlowBusLib/Load Flow Bus  LConnTagsString=a  Phases=single  Connectors=on one side  ID=BUS_12  Vbase=230e3  Vref=1.055  Vangle=0  VLF=0.9418  VLFb=1  VLFc=1  angleLF=-36.13  angleLFb=0  angleLFc=0
  Load Flow Bus14 : spsLoadFlowBusLib/Load Flow Bus  LConnTagsString=a  Phases=single  Connectors=on one side  ID=BUS_14  Vbase=230e3  Vref=1.036  Vangle=0  VLF=0.9414  VLFb=1  VLFc=1  angleLF=-36.19  angleLFb=0  angleLFc=0
  Load Flow Bus15 : spsLoadFlowBusLib/Load Flow Bus  LConnTagsString=a  Phases=single  Connectors=on one side  ID=BUS_c  Vbase=139.38e3  Vref=1.010  Vangle=0  VLF=0.9282  VLFb=1  VLFc=1  angleLF=-34.24  angleLFb=0  angleLFc=0
  Load Flow Bus16 : spsLoadFlowBusLib/Load Flow Bus  LConnTagsString=a  Phases=single  Connectors=on one side  ID=BUS_a  Vbase=146.28e3  Vref=1.0  Vangle=0  VLF=0.9625  VLFb=1  VLFc=1  angleLF=-19.37  angleLFb=0  angleLFc=0
  Load Flow Bus17 : spsLoadFlowBusLib/Load Flow Bus  LConnTagsString=a  Phases=single  Connectors=on one side  ID=BUS_b  Vbase=144.21e3  Vref=1.045  Vangle=0  VLF=0.9497  VLFb=1  VLFc=1  angleLF=-24.42  angleLFb=0  angleLFc=0
  Load Flow Bus18 : spsLoadFlowBusLib/Load Flow Bus  LConnTagsString=a  Phases=single  Connectors=on one side  ID=BUS_d  Vbase=147.66e3  Vref=1.070  Vangle=0  VLF=0.9625  VLFb=1  VLFc=1  angleLF=-19.37  angleLFb=0  angleLFc=0
  Load Flow Bus19 : spsLoadFlowBusLib/Load Flow Bus  LConnTagsString=a  Phases=single  Connectors=on one side  ID=BUS_e  Vbase=150.420e3  Vref=1.090  Vangle=0  VLF=0.9461  VLFb=1  VLFc=1  angleLF=-36  angleLFb=0  angleLFc=0
  Load Flow Bus2 : spsLoadFlowBusLib/Load Flow Bus  LConnTagsString=a  Phases=single  Connectors=on one side  ID=BUS_7  Vbase=230e3  Vref=1.062  Vangle=0  VLF=0.9439  VLFb=1  VLFc=1  angleLF=-36  angleLFb=0  angleLFc=0
  Load Flow Bus20 : spsLoadFlowBusLib/Load Flow Bus  LConnTagsString=a  Phases=single  Connectors=on one side  ID=1  Vbase=10e3  Vref=1.06  Vangle=0  VLF=1.06  VLFb=1  VLFc=1  angleLF=0  angleLFb=0  angleLFc=0
  Load Flow Bus21 : spsLoadFlowBusLib/Load Flow Bus  LConnTagsString=a  Phases=single  Connectors=on one side  ID=11  Vbase=10e3  Vref=1  Vangle=0  VLF=1.047  VLFb=1  VLFc=1  angleLF=-2.806  angleLFb=0  angleLFc=0
  Load Flow Bus22 : spsLoadFlowBusLib/Load Flow Bus  LConnTagsString=a  Phases=single  Connectors=on one side  ID=12  Vbase=10e3  Vref=1  Vangle=0  VLF=1.047  VLFb=1  VLFc=1  angleLF=-2.806  angleLFb=0  angleLFc=0
  Load Flow Bus23 : spsLoadFlowBusLib/Load Flow Bus  LConnTagsString=a  Phases=single  Connectors=on one side  ID=13  Vbase=10e3  Vref=1  Vangle=0  VLF=1.047  VLFb=1  VLFc=1  angleLF=-2.806  angleLFb=0  angleLFc=0
  Load Flow Bus24 : spsLoadFlowBusLib/Load Flow Bus  LConnTagsString=a  Phases=single  Connectors=on one side  ID=14  Vbase=10e3  Vref=1  Vangle=0  VLF=1.047  VLFb=1  VLFc=1  angleLF=-2.806  angleLFb=0  angleLFc=0
  Load Flow Bus25 : spsLoadFlowBusLib/Load Flow Bus  LConnTagsString=a  Phases=single  Connectors=on one side  ID=5  Vbase=10e3  Vref=1  Vangle=0  VLF=1.06  VLFb=1  VLFc=1  angleLF=0  angleLFb=0  angleLFc=0
  Load Flow Bus26 : spsLoadFlowBusLib/Load Flow Bus  LConnTagsString=a  Phases=single  Connectors=on one side  ID=2  Vbase=10e3  Vref=1.045  Vangle=0  VLF=1.06  VLFb=1  VLFc=1  angleLF=0  angleLFb=0  angleLFc=0
  Load Flow Bus27 : spsLoadFlowBusLib/Load Flow Bus  LConnTagsString=a  Phases=single  Connectors=on one side  ID=3  Vbase=10e3  Vref=1.01  Vangle=0  VLF=1.06  VLFb=1  VLFc=1  angleLF=0  angleLFb=0  angleLFc=0
  Load Flow Bus28 : spsLoadFlowBusLib/Load Flow Bus  LConnTagsString=a  Phases=single  Connectors=on one side  ID=4  Vbase=10e3  Vref=1  Vangle=0  VLF=1.06  VLFb=1  VLFc=1  angleLF=0  angleLFb=0  angleLFc=0
  Load Flow Bus29 : spsLoadFlowBusLib/Load Flow Bus  LConnTagsString=a  Phases=single  Connectors=on one side  ID=7  Vbase=10e3  Vref=1  Vangle=0  VLF=1.047  VLFb=1  VLFc=1  angleLF=-2.806  angleLFb=0  angleLFc=0
  Load Flow Bus3 : spsLoadFlowBusLib/Load Flow Bus  LConnTagsString=a  Phases=single  Connectors=on one side  ID=BUS_8  Vbase=230e3  Vref=1.090  Vangle=0  VLF=0.9461  VLFb=1  VLFc=1  angleLF=-36  angleLFb=0  angleLFc=0
  Load Flow Bus30 : spsLoadFlowBusLib/Load Flow Bus  LConnTagsString=a  Phases=single  Connectors=on one side  ID=6  Vbase=10e3  Vref=1.07  Vangle=0  VLF=1.06  VLFb=1  VLFc=1  angleLF=0  angleLFb=0  angleLFc=0
  Load Flow Bus31 : spsLoadFlowBusLib/Load Flow Bus  LConnTagsString=a  Phases=single  Connectors=on one side  ID=10  Vbase=10e3  Vref=1  Vangle=0  VLF=1.047  VLFb=1  VLFc=1  angleLF=-2.806  angleLFb=0  angleLFc=0
  Load Flow Bus32 : spsLoadFlowBusLib/Load Flow Bus  LConnTagsString=a  Phases=single  Connectors=on one side  ID=8  Vbase=10e3  Vref=1.09  Vangle=0  VLF=1.047  VLFb=1  VLFc=1  angleLF=-2.806  angleLFb=0  angleLFc=0
  Load Flow Bus33 : spsLoadFlowBusLib/Load Flow Bus  LConnTagsString=a  Phases=single  Connectors=on one side  ID=9  Vbase=10e3  Vref=1  Vangle=0  VLF=1.047  VLFb=1  VLFc=1  angleLF=-2.806  angleLFb=0  angleLFc=0
  Load Flow Bus4 : spsLoadFlowBusLib/Load Flow Bus  LConnTagsString=a  Phases=single  Connectors=on one side  ID=BUS_3  Vbase=230e3  Vref=1.010  Vangle=0  VLF=0.9282  VLFb=1  VLFc=1  angleLF=-34.24  angleLFb=0  angleLFc=0
  Load Flow Bus5 : spsLoadFlowBusLib/Load Flow Bus  LConnTagsString=a  Phases=single  Connectors=on one side  ID=BUS_10  Vbase=230e3  Vref=1.051  Vangle=0  VLF=0.9425  VLFb=1  VLFc=1  angleLF=-36.13  angleLFb=0  angleLFc=0
  Load Flow Bus6 : spsLoadFlowBusLib/Load Flow Bus  LConnTagsString=a  Phases=single  Connectors=on one side  ID=BUS_2  Vbase=230e3  Vref=1.045  Vangle=0  VLF=0.9497  VLFb=1  VLFc=1  angleLF=-24.42  angleLFb=0  angleLFc=0
  Load Flow Bus7 : spsLoadFlowBusLib/Load Flow Bus  LConnTagsString=a  Phases=single  Connectors=on one side  ID=BUS_11  Vbase=230e3  Vref=1.057  Vangle=0  VLF=0.9423  VLFb=1  VLFc=1  angleLF=-36.11  angleLFb=0  angleLFc=0
  Load Flow Bus8 : spsLoadFlowBusLib/Load Flow Bus  LConnTagsString=a  Phases=single  Connectors=on one side  ID=BUS_9  Vbase=230e3  Vref=1.056  Vangle=0  VLF=0.943  VLFb=1  VLFc=1  angleLF=-36.12  angleLFb=0  angleLFc=0
  Load Flow Bus9 : spsLoadFlowBusLib/Load Flow Bus  LConnTagsString=a  Phases=single  Connectors=on one side  ID=BUS_5  Vbase=230e3  Vref=1.020  Vangle=0  VLF=0.9312  VLFb=1  VLFc=1  angleLF=-29.41  angleLFb=0  angleLFc=0
  SWING 1 : spsThreePhaseSourceLib/Three-Phase Source  InternalConnection=Yg  VoltagePhases=off  Voltage=(10000)*1.06  PhaseAngle=0  Voltage_phases=[25e3 25e3 25e3]/sqrt(3)  PhaseAngles_phases=[0 -120 +120]  Frequency=60  NonIdealSource=off  SpecifyImpedance=off  Resistance=0.8929  Inductance=16.58e-3  ShortCircuitLevel=100e6  BaseVoltage=25e3  XRratio=7  BusType=swing  Pref=10e3  Qref=0  Prefabc=[10e3, 10e3, 10e3]  Qrefabc=[0, 0, 0]  Qmin=0  Qmax=0
  Synchronous condensor_1 : spsThreePhaseSourceLib/Three-Phase Source  InternalConnection=Yg  VoltagePhases=off  Voltage=(139380)*1.010  PhaseAngle=-34.48  Voltage_phases=[25e3 25e3 25e3]/sqrt(3)  PhaseAngles_phases=[0 -120 +120]  Frequency=60  NonIdealSource=on  SpecifyImpedance=off  Resistance=0.8929  Inductance=16.58e-3  ShortCircuitLevel=100e6  BaseVoltage=139.38e3  XRratio=7  BusType=PV  Pref=0  Qref=50.096e6  Prefabc=[10e3, 10e3, 10e3]  Qrefabc=[0, 0, 0]  Qmin=0  Qmax=40e6
  Synchronous condensor_2 : spsThreePhaseSourceLib/Three-Phase Source  InternalConnection=Yg  VoltagePhases=off  Voltage=(147660)*1.070  PhaseAngle=-36.2022  Voltage_phases=[25e3 25e3 25e3]/sqrt(3)  PhaseAngles_phases=[0 -120 +120]  Frequency=60  NonIdealSource=on  SpecifyImpedance=off  Resistance=0.8929  Inductance=16.58e-3  ShortCircuitLevel=100e6  BaseVoltage=147.66e3  XRratio=7  BusType=PV  Pref=0  Qref=25.276e6  Prefabc=[10e3, 10e3, 10e3]  Qrefabc=[0, 0, 0]  Qmin=-6e6  Qmax=24e6
  Synchronous condensor_3 : spsThreePhaseSourceLib/Three-Phase Source  InternalConnection=Yg  VoltagePhases=off  Voltage=(150420)*1.090  PhaseAngle=-36.1424  Voltage_phases=[25e3 25e3 25e3]/sqrt(3)  PhaseAngles_phases=[0 -120 +120]  Frequency=60  NonIdealSource=on  SpecifyImpedance=off  Resistance=0.8929  Inductance=16.58e-3  ShortCircuitLevel=100e6  BaseVoltage=150.42e3  XRratio=7  BusType=PV  Pref=0  Qref=30.144e6  Prefabc=[10e3, 10e3, 10e3]  Qrefabc=[0, 0, 0]  Qmin=-6e6  Qmax=24e6
  Three-Phase Series RLC Load : spsThreePhaseSeriesRLCLoadLib/Three-Phase Series RLC Load  LConnTagsString=A|B|C  Configuration=Y (grounded)  NominalVoltage=(230000)*1.045  Vabc=[1e3 1e3 1e3]  Vabcp=[1e3 1e3 1e3]  NominalFrequency=60  UnbalancedPower=off  ActivePower=26.04e6  InductivePower=15.24e6  CapacitivePower=0  Pabc=[10e3 9e3 11e3]  QLabc=[100 90 110]  QCabc=[100 90 110]  Pabcp=[10e3 9e3 11e3]  QLabcp=[100 90 110]  QCabcp=[100 90 110]  Measurements=None  LoadType=constant PQ
  Three-Phase Series RLC Load1 : spsThreePhaseSeriesRLCLoadLib/Three-Phase Series RLC Load  LConnTagsString=A|B|C  Configuration=Y (grounded)  NominalVoltage=(230000)*0.92821  Vabc=[1e3 1e3 1e3]  Vabcp=[1e3 1e3 1e3]  NominalFrequency=60  UnbalancedPower=off  ActivePower=113.04e6  InductivePower=22.8e6  CapacitivePower=0  Pabc=[10e3 9e3 11e3]  QLabc=[100 90 110]  QCabc=[100 90 110]  Pabcp=[10e3 9e3 11e3]  QLabcp=[100 90 110]  QCabcp=[100 90 110]  Measurements=None  LoadType=constant PQ
  Three-Phase Series RLC Load10 : spsThreePhaseSeriesRLCLoadLib/Three-Phase Series RLC Load  LConnTagsString=A|B|C  Configuration=Y (grounded)  NominalVoltage=(230000)*0.942986  Vabc=[1e3 1e3 1e3]  Vabcp=[1e3 1e3 1e3]  NominalFrequency=60  UnbalancedPower=off  ActivePower=35.4e6  InductivePower=19.92e6  CapacitivePower=0  Pabc=[10e3 9e3 11e3]  QLabc=[100 90 110]  QCabc=[100 90 110]  Pabcp=[10e3 9e3 11e3]  QLabcp=[100 90 110]  QCabcp=[100 90 110]  Measurements=None  LoadType=constant PQ
  Three-Phase Series RLC Load2 : spsThreePhaseSeriesRLCLoadLib/Three-Phase Series RLC Load  LConnTagsString=A|B|C  Configuration=Y (grounded)  NominalVoltage=(230000)*0.927953  Vabc=[1e3 1e3 1e3]  Vabcp=[1e3 1e3 1e3]  NominalFrequency=60  UnbalancedPower=off  ActivePower=57.36e6  InductivePower=0  CapacitivePower=4.68e6  Pabc=[10e3 9e3 11e3]  QLabc=[100 90 110]  QCabc=[100 90 110]  Pabcp=[10e3 9e3 11e3]  QLabcp=[100 90 110]  QCabcp=[100 90 110]  Measurements=None  LoadType=constant PQ
  Three-Phase Series RLC Load3 : spsThreePhaseSeriesRLCLoadLib/Three-Phase Series RLC Load  LConnTagsString=A|B|C  Configuration=Y (grounded)  NominalVoltage=(230000)*0.931217  Vabc=[1e3 1e3 1e3]  Vabcp=[1e3 1e3 1e3]  NominalFrequency=60  UnbalancedPower=off  ActivePower=9.12e6  InductivePower=1.92e6  CapacitivePower=0  Pabc=[10e3 9e3 11e3]  QLabc=[100 90 110]  QCabc=[100 90 110]  Pabcp=[10e3 9e3 11e3]  QLabcp=[100 90 110]  QCabcp=[100 90 110]  Measurements=None  LoadType=constant PQ
  Three-Phase Series RLC Load4 : spsThreePhaseSeriesRLCLoadLib/Three-Phase Series RLC Load  LConnTagsString=A|B|C  Configuration=Y (grounded)  NominalVoltage=(230000)*0.942548  Vabc=[1e3 1e3 1e3]  Vabcp=[1e3 1e3 1e3]  NominalFrequency=60  UnbalancedPower=off  ActivePower=13.44e6  InductivePower=9e6  CapacitivePower=0  Pabc=[10e3 9e3 11e3]  QLabc=[100 90 110]  QCabc=[100 90 110]  Pabcp=[10e3 9e3 11e3]  QLabcp=[100 90 110]  QCabcp=[100 90 110]  Measurements=None  LoadType=constant PQ
  Three-Phase Series RLC Load5 : spsThreePhaseSeriesRLCLoadLib/Three-Phase Series RLC Load  LConnTagsString=A|B|C  Configuration=Y (grounded)  NominalVoltage=(230000)*0.942502  Vabc=[1e3 1e3 1e3]  Vabcp=[1e3 1e3 1e3]  NominalFrequency=60  UnbalancedPower=off  ActivePower=10.8e6  InductivePower=6.96e6  CapacitivePower=0  Pabc=[10e3 9e3 11e3]  QLabc=[100 90 110]  QCabc=[100 90 110]  Pabcp=[10e3 9e3 11e3]  QLabcp=[100 90 110]  QCabcp=[100 90 110]  Measurements=None  LoadType=constant PQ
  Three-Phase Series RLC Load6 : spsThreePhaseSeriesRLCLoadLib/Three-Phase Series RLC Load  LConnTagsString=A|B|C  Configuration=Y (grounded)  NominalVoltage=(230000)*0.942338  Vabc=[1e3 1e3 1e3]  Vabcp=[1e3 1e3 1e3]  NominalFrequency=60  UnbalancedPower=off  ActivePower=4.2e6  InductivePower=2.16e6  CapacitivePower=0  Pabc=[10e3 9e3 11e3]  QLabc=[100 90 110]  QCabc=[100 90 110]  Pabcp=[10e3 9e3 11e3]  QLabcp=[100 90 110]  QCabcp=[100 90 110]  Measurements=None  LoadType=constant PQ
  Three-Phase Series RLC Load7 : spsThreePhaseSeriesRLCLoadLib/Three-Phase Series RLC Load  LConnTagsString=A|B|C  Configuration=Y (grounded)  NominalVoltage=(230000)*0.941818  Vabc=[1e3 1e3 1e3]  Vabcp=[1e3 1e3 1e3]  NominalFrequency=60  UnbalancedPower=off  ActivePower=7.32e6  InductivePower=1.92e6  CapacitivePower=0  Pabc=[10e3 9e3 11e3]  QLabc=[100 90 110]  QCabc=[100 90 110]  Pabcp=[10e3 9e3 11e3]  QLabcp=[100 90 110]  QCabcp=[100 90 110]  Measurements=None  LoadType=constant PQ
  Three-Phase Series RLC Load8 : spsThreePhaseSeriesRLCLoadLib/Three-Phase Series RLC Load  LConnTagsString=A|B|C  Configuration=Y (grounded)  NominalVoltage=(230000)*0.941642  Vabc=[1e3 1e3 1e3]  Vabcp=[1e3 1e3 1e3]  NominalFrequency=60  UnbalancedPower=off  ActivePower=16.2e6  InductivePower=6.96e6  CapacitivePower=0  Pabc=[10e3 9e3 11e3]  QLabc=[100 90 110]  QCabc=[100 90 110]  Pabcp=[10e3 9e3 11e3]  QLabcp=[100 90 110]  QCabcp=[100 90 110]  Measurements=None  LoadType=constant PQ
  Three-Phase Series RLC Load9 : spsThreePhaseSeriesRLCLoadLib/Three-Phase Series RLC Load  LConnTagsString=A|B|C  Configuration=Y (grounded)  NominalVoltage=(230000)*0.941422  Vabc=[1e3 1e3 1e3]  Vabcp=[1e3 1e3 1e3]  NominalFrequency=60  UnbalancedPower=off  ActivePower=17.88e6  InductivePower=6e6  CapacitivePower=0  Pabc=[10e3 9e3 11e3]  QLabc=[100 90 110]  QCabc=[100 90 110]  Pabcp=[10e3 9e3 11e3]  QLabcp=[100 90 110]  QCabcp=[100 90 110]  Measurements=None  LoadType=constant PQ
  powergui : spspowerguiLib/powergui  Priority=1  SimulationMode=Discrete  SampleTime=50e-6  frequency=60  Iterations=50  frequencyindice=60  Pbase=120e6  ErrMax=0.0001  UnitsV=kV  UnitsW=MW  buscounter=0  FunctionMessages=off  echomessages=off  EnableUseOfTLC=off  CurrentSourceSwitches=off  DisableSnubberDevices=off  DisableRonSwitches=off  DisableVfSwitches=off  DisplayEquations=off  AutomaticDiscreteSolvers=off  SolverType=Tustin/Backward Euler (TBE)  Interpol=off  ExternalGateDelay=off  methode=off  Ts=100  x0status=blocks  SPID=on  SwTol=0  HookPort=off  NonlinearTolerance=1e-4  nMaxIteration=500  ContinueOnMaxIteration=off  RestoreLinks=warning  ResistiveCurrentMeasurement=off  Frange=[0:2:500]  Ylog=off  Xlog=on  ShowGrid=off  save=off  variable=ZData  structure=0  ZoomFFT=off  StartTime=0.0  cycles=1  DisplayStyle=1  fundamental=60  FreqAxis=off  MaxFrequency=1000  frequencyindicesteady=1  RmsSteady=1  display=off
  powergui1 : spspowerguiLib/powergui  Priority=1  SimulationMode=Continuous  SampleTime=50e-6  frequency=60  Iterations=50  frequencyindice=60  Pbase=100e6  ErrMax=1e-4  UnitsV=kV  UnitsW=MW  buscounter=0  FunctionMessages=off  echomessages=off  EnableUseOfTLC=off  CurrentSourceSwitches=off  DisableSnubberDevices=off  DisableRonSwitches=off  DisableVfSwitches=off  DisplayEquations=off  AutomaticDiscreteSolvers=off  SolverType=Tustin/Backward Euler (TBE)  Interpol=off  ExternalGateDelay=off  methode=off  Ts=100  x0status=blocks  SPID=on  SwTol=0  HookPort=off  NonlinearTolerance=1e-4  nMaxIteration=100  ContinueOnMaxIteration=off  RestoreLinks=warning  ResistiveCurrentMeasurement=off  Frange=[0:2:500]  Ylog=off  Xlog=on  ShowGrid=off  save=off  variable=ZData  structure=0  ZoomFFT=off  StartTime=0.0  cycles=1  DisplayStyle=1  fundamental=60  FreqAxis=off  MaxFrequency=1000  frequencyindicesteady=1  RmsSteady=1  display=off
  connections:
  146.28/230kV/LConn1 -- Generator 1/RConn1
  146.28/230kV/RConn1 -- Bus_1/LConn3
  146.28/230kV/RConn2 -- Bus_1/LConn2
  146.28/230kV/RConn3 -- Load Flow Bus10/LConn1 -- Bus_1/LConn1
  Generator 1/RConn2 -- 146.28/230kV/LConn2
  Generator 1/RConn3 -- Load Flow Bus16/LConn1 -- 146.28/230kV/LConn3
  Bus_2/RConn4 -- 144.21/230kV/RConn1
  144.21/230kV/LConn1 -- Load Flow Bus17/LConn1 -- Generator 2/RConn1
  Bus_2/RConn5 -- 144.21/230kV/RConn2
  Generator 2/RConn2 -- 144.21/230kV/LConn2
  Generator 2/RConn3 -- 144.21/230kV/LConn3
  Bus_2/LConn1 -- Line 1-2/RConn1 -- Load Flow Bus6/LConn1
  Line 1-2/LConn3 -- Bus_1/RConn3
  Line 1-2/LConn2 -- Bus_1/RConn2
  Line 1-2/LConn1 -- Bus_1/RConn1
  Line 1-2/RConn2 -- Bus_2/LConn2
  Line 1-2/RConn3 -- Bus_2/LConn3
  Line 2-4/LConn1 -- Bus_2/LConn7
  Line 2-4/LConn2 -- Bus_2/LConn8
  Line 2-4/LConn3 -- Bus_2/LConn9
  Line 2-3/RConn3 -- Bus_3/RConn3
  Line 2-3/RConn2 -- Bus_3/RConn2
  Line 2-3/RConn1 -- Bus_3/RConn1
  Bus_3/RConn9 -- 139.38/230kV/RConn3 -- Load Flow Bus4/LConn1
  Synchronous condensor_1/RConn3 -- 139.38/230kV/LConn3 -- Load Flow Bus15/LConn1
  Bus_3/RConn7 -- 139.38/230kV/RConn1
  Synchronous condensor_1/RConn2 -- 139.38/230kV/LConn2
  139.38/230kV/LConn1 -- Synchronous condensor_1/RConn1
  Bus_3/RConn8 -- 139.38/230kV/RConn2
  Line 3-4/RConn2 -- Bus_3/LConn2
  Line 3-4/RConn3 -- Bus_3/LConn3
  Line 3-4/RConn1 -- Bus_3/LConn1
  Line 3-4/LConn3 -- Bus_4/RConn9
  Line 3-4/LConn2 -- Bus_4/RConn8
  Line 3-4/LConn1 -- Bus_4/RConn7
  Line 2-4/RConn1 -- Bus_4/RConn4
  Line 2-4/RConn2 -- Bus_4/RConn5
  Line 2-4/RConn3 -- Bus_4/RConn6
  Line 4-5/RConn1 -- Bus_4/RConn1
  Line 4-5/RConn2 -- Bus_4/RConn2
  Line 4-5/RConn3 -- Bus_4/RConn3
  Line 4-5/LConn1 -- Bus_5/RConn9
  Line 4-5/LConn2 -- Bus_5/RConn8
  Line 4-5/LConn3 -- Bus_5/RConn7
  Line 1-5/RConn1 -- Bus_5/RConn1
  Line 1-5/RConn2 -- Bus_5/RConn2
  Line 1-5/RConn3 -- Bus_5/RConn3
  Bus_1/RConn6 -- Line 1-5/LConn1
  Bus_1/RConn5 -- Line 1-5/LConn2
  Bus_1/RConn4 -- Line 1-5/LConn3
  Line 5-6/RConn2 -- Bus_5/LConn5
  Load Flow Bus9/LConn1 -- Line 5-6/RConn3 -- Bus_5/LConn6
  Line 5-6/RConn1 -- Bus_5/LConn4
  Line 5-6/LConn2 -- Bus_6/LConn5
  Bus_6/LConn6 -- Line 5-6/LConn3 -- Load Flow Bus11/LConn1
  Line 5-6/LConn1 -- Bus_6/LConn4
  Synchronous condensor_2/RConn3 -- Load Flow Bus18/LConn1 -- 147.66/230kV/LConn3
  Synchronous condensor_2/RConn1 -- 147.66/230kV/LConn1
  Synchronous condensor_2/RConn2 -- 147.66/230kV/LConn2
  147.66/230kV/RConn1 -- Bus_6/LConn1
  147.66/230kV/RConn2 -- Bus_6/LConn2
  147.66/230kV/RConn3 -- Bus_6/LConn3
  Line 6-13/RConn1 -- Bus_6/RConn4
  Line 6-13/RConn2 -- Bus_6/RConn5
  Line 6-13/RConn3 -- Bus_6/RConn6
  Line 6-12/RConn3 -- Bus_6/RConn3
  Line 6-12/RConn1 -- Bus_6/RConn1
  Line 6-12/RConn2 -- Bus_6/RConn2
  Bus_12/RConn1 -- Line 6-12/LConn1 -- Load Flow Bus13/LConn1
  Line 6-12/LConn2 -- Bus_12/RConn2
  Line 6-12/LConn3 -- Bus_12/RConn3
  Line 12-13/LConn1 -- Bus_12/RConn6
  Line 12-13/LConn2 -- Bus_12/RConn5
  Line 12-13/LConn3 -- Bus_12/RConn4
  Line 6-13/LConn1 -- Bus_13/RConn4
  Line 6-13/LConn2 -- Bus_13/RConn5
  Line 6-13/LConn3 -- Bus_13/RConn6
  Line 12-13/RConn1 -- Bus_13/RConn1
  Line 12-13/RConn2 -- Bus_13/RConn2
  Line 12-13/RConn3 -- Bus_13/RConn3
  Load Flow Bus12/LConn1 -- Three-Phase Series RLC Load8/LConn3 -- Bus_13/LConn3
  Line 13-14/LConn1 -- Bus_13/RConn9
  Line 13-14/LConn2 -- Bus_13/RConn8
  Line 13-14/LConn3 -- Bus_13/RConn7
  Line 13-14/RConn1 -- Bus_14/RConn1
  Line 13-14/RConn2 -- Bus_14/RConn2
  Line 13-14/RConn3 -- Bus_14/RConn3
  Line 6-11/RConn1 -- Bus_11/RConn1
  Line 6-11/RConn2 -- Bus_11/RConn2
  Line 6-11/RConn3 -- Bus_11/RConn3
  Line 6-11/LConn1 -- Bus_6/RConn7
  Line 6-11/LConn2 -- Bus_6/RConn8
  Line 6-11/LConn3 -- Bus_6/RConn9
  Load Flow Bus7/LConn1 -- Three-Phase Series RLC Load6/LConn3 -- Bus_11/LConn3
  Line 10-11/LConn1 -- Bus_11/RConn6
  Line 10-11/LConn2 -- Bus_11/RConn5
  Line 10-11/LConn3 -- Bus_11/RConn4
  Line 10-11/RConn1 -- Bus_10/RConn1
  Line 10-11/RConn2 -- Bus_10/RConn2
  Line 10-11/RConn3 -- Bus_10/RConn3
  Line 9-10/LConn1 -- Bus_10/RConn6
  Line 9-10/LConn2 -- Bus_10/RConn5
  Line 9-10/LConn3 -- Bus_10/RConn4
  Load Flow Bus5/LConn1 -- Three-Phase Series RLC Load5/LConn3 -- Bus_10/LConn3
  Load Flow Bus14/LConn1 -- Three-Phase Series RLC Load9/LConn3 -- Bus_14/LConn3
  Line 9-10/RConn1 -- Bus_9/RConn1
  Line 9-10/RConn2 -- Bus_9/RConn2
  Line 9-10/RConn3 -- Bus_9/RConn3
  Line 9-14/RConn2 -- Bus_9/LConn2
  Bus_9/LConn1 -- Line 9-14/RConn1 -- Load Flow Bus8/LConn1
  Line 9-14/RConn3 -- Bus_9/LConn3
  Line 9-14/LConn1 -- Bus_14/RConn4
  Line 9-14/LConn2 -- Bus_14/RConn5
  Line 9-14/LConn3 -- Bus_14/RConn6
  Line 4-9/RConn2 -- Bus_4/LConn2
  Line 4-9/RConn1 -- Bus_4/LConn1
  Line 4-9/RConn3 -- Bus_4/LConn3
  Line 4-9/LConn1 -- Bus_9/RConn4
  Line 4-9/LConn2 -- Bus_9/RConn5
  Line 4-9/LConn3 -- Bus_9/RConn6
  Line 4-7/RConn2 -- Bus_4/LConn5
  Line 4-7/RConn1 -- Bus_4/LConn4
  Bus_4/LConn6 -- Line 4-7/RConn3 -- Load Flow Bus1/LConn1
  Line 4-7/LConn2 -- Bus_7/LConn2
  Line 4-7/LConn1 -- Bus_7/LConn1
  Line 4-7/LConn3 -- Bus_7/LConn3
  Line 7-9/RConn1 -- Bus_7/RConn1
  Line 7-9/RConn2 -- Bus_7/RConn2
  Line 7-9/RConn3 -- Bus_7/RConn3
  Line 7-9/LConn1 -- Bus_9/RConn7
  Line 7-9/LConn2 -- Bus_9/RConn8
  Line 7-9/LConn3 -- Bus_9/RConn9
  Load Flow Bus2/LConn1 -- Line 7-8/LConn3 -- Bus_7/RConn6
  Line 7-8/LConn2 -- Bus_7/RConn5
  Line 7-8/LConn1 -- Bus_7/RConn4
  150.42/230kV/RConn2 -- Bus_8/RConn2
  Line 7-8/RConn1 -- Bus_8/LConn1
  Line 7-8/RConn2 -- Bus_8/LConn2
  Line 7-8/RConn3 -- Bus_8/LConn3
  Bus_8/RConn1 -- Load Flow Bus3/LConn1 -- 150.42/230kV/RConn1
  150.42/230kV/RConn3 -- Bus_8/RConn3
  Synchronous condensor_3/RConn2 -- 150.42/230kV/LConn2
  Synchronous condensor_3/RConn3 -- Load Flow Bus19/LConn1 -- 150.42/230kV/LConn3
  Synchronous condensor_3/RConn1 -- 150.42/230kV/LConn1
  Bus_2/RConn6 -- 144.21/230kV/RConn3
  Line 2-3/LConn1 -- Bus_2/RConn9
  Line 2-3/LConn2 -- Bus_2/RConn8
  Line 2-3/LConn3 -- Bus_2/RConn7
  Line 2-5/RConn2 -- Bus_5/RConn5
  Line 2-5/LConn2 -- Bus_2/LConn5
  Line 2-5/LConn1 -- Bus_2/LConn6
  Line 2-5/LConn3 -- Bus_2/LConn4
  Line 2-5/RConn3 -- Bus_5/RConn4
  Line 2-5/RConn1 -- Bus_5/RConn6
  " "/LConn1 -- Bus_9/LConn4
  " "/LConn2 -- Bus_9/LConn5
  " "/LConn3 -- Bus_9/LConn6
  Three-Phase Series RLC Load/LConn3 -- Bus_2/RConn3
  Three-Phase Series RLC Load/LConn2 -- Bus_2/RConn2
  Three-Phase Series RLC Load/LConn1 -- Bus_2/RConn1
  Three-Phase Series RLC Load1/LConn3 -- Bus_3/RConn6
  Three-Phase Series RLC Load1/LConn2 -- Bus_3/RConn5
  Three-Phase Series RLC Load1/LConn1 -- Bus_3/RConn4
  Three-Phase Series RLC Load3/LConn1 -- Bus_5/LConn3
  Three-Phase Series RLC Load3/LConn2 -- Bus_5/LConn2
  Three-Phase Series RLC Load3/LConn3 -- Bus_5/LConn1
  Three-Phase Series RLC Load10/LConn1 -- Bus_9/RConn12
  Three-Phase Series RLC Load10/LConn2 -- Bus_9/RConn11
  Three-Phase Series RLC Load10/LConn3 -- Bus_9/RConn10
  Three-Phase Series RLC Load6/LConn2 -- Bus_11/LConn2
  Three-Phase Series RLC Load6/LConn1 -- Bus_11/LConn1
  Three-Phase Series RLC Load7/LConn3 -- Bus_12/LConn3
  Three-Phase Series RLC Load7/LConn2 -- Bus_12/LConn2
  Three-Phase Series RLC Load7/LConn1 -- Bus_12/LConn1
  Three-Phase Series RLC Load8/LConn2 -- Bus_13/LConn2
  Three-Phase Series RLC Load8/LConn1 -- Bus_13/LConn1
  Three-Phase Series RLC Load9/LConn1 -- Bus_14/LConn1
  Three-Phase Series RLC Load9/LConn2 -- Bus_14/LConn2
  Three-Phase Series RLC Load2/LConn1 -- Bus_4/RConn10
  Three-Phase Series RLC Load2/LConn2 -- Bus_4/RConn11
  Three-Phase Series RLC Load2/LConn3 -- Bus_4/RConn12
  Three-Phase Series RLC Load5/LConn1 -- Bus_10/LConn1
  Three-Phase Series RLC Load5/LConn2 -- Bus_10/LConn2
  Three-Phase Series RLC Load4/LConn1 -- Bus_6/RConn10
  Three-Phase Series RLC Load4/LConn2 -- Bus_6/RConn11
  Three-Phase Series RLC Load4/LConn3 -- Bus_6/RConn12
  BUS 9/LConn2 -- Line 9-2/RConn2 -- Line 4-3/LConn2 -- Line 9-1/RConn2 -- Line 7-2/LConn2
  Line 9-1/RConn1 -- Line 4-3/LConn1 -- Line 7-2/LConn1 -- Line 9-2/RConn1 -- BUS 9/LConn1
  BUS 7/LConn3 -- Line 4-2/LConn3 -- Line 7-1/RConn3 -- Line 7-2/RConn3
  LOAD 9/LConn2 -- " 1"/LConn2 -- BUS 9/RConn2
  Line 6-3/LConn2 -- BUS 13/LConn2 -- Line 13-1/LConn2 -- Line 12-1/LConn2
  Line 9-2/LConn3 -- BUS 14/LConn3 -- Line 13-1/RConn3
  Line 6-3/LConn3 -- BUS 13/LConn3 -- Line 13-1/LConn3 -- Line 12-1/LConn3
  Line 6-1/LConn3 -- BUS 11/LConn3 -- Line 10-1/RConn3
  Load Flow Bus24/LConn1 -- LOAD 14/LConn1 -- BUS 14/RConn1
  BUS 3/RConn3 -- Line 2-1/RConn3 -- Line 3-1/LConn3
  BUS 2/LConn3 -- LOAD 2/LConn3 -- GEN 2/RConn3
  Line 12-1/RConn3 -- BUS 12/LConn3 -- Line 6-2/LConn3
  GEN 6/RConn1 -- LOAD 6/LConn1 -- BUS 6/RConn1 -- Load Flow Bus30/LConn1
  BUS 9/LConn3 -- Line 4-3/LConn3 -- Line 9-1/RConn3 -- Line 7-2/LConn3 -- Line 9-2/RConn3
  BUS 3/LConn3 -- LOAD 3/LConn3 -- GEN 3/RConn3
  Line 2-2/RConn1 -- Line 3-1/RConn1 -- Line 4-1/RConn1 -- Line 4-2/RConn1 -- BUS 4/LConn1 -- Line 4-3/RConn1
  Line 6-1/LConn2 -- BUS 11/LConn2 -- Line 10-1/RConn2
  Line 1-1/LConn2 -- BUS 1/RConn2 -- Line 1-3/LConn2
  Line 9-2/LConn2 -- BUS 14/LConn2 -- Line 13-1/RConn2
  BUS 6/LConn3 -- Line 6-1/RConn3 -- Line 5-1/RConn3 -- Line 6-3/RConn3 -- Line 6-2/RConn3
  Load Flow Bus29/LConn1 -- BUS 7/LConn1 -- Line 4-2/LConn1 -- Line 7-1/RConn1 -- Line 7-2/RConn1
  Line 2-2/LConn1 -- Line 1-1/RConn1 -- Line 2-1/LConn1 -- BUS 2/RConn1 -- Line 2-6/RConn1
  Line 6-2/LConn2 -- BUS 12/LConn2 -- Line 12-1/RConn2
  BUS 6/LConn2 -- Line 5-1/RConn2 -- Line 6-3/RConn2 -- Line 6-2/RConn2 -- Line 6-1/RConn2
  Line 9-1/LConn2 -- BUS 10/LConn2 -- Line 10-1/LConn2
  Line 1-3/RConn1 -- Line 2-6/LConn1 -- Line 5-1/LConn1 -- BUS 5/LConn1 -- Load Flow Bus25/LConn1 -- Line 4-1/LConn1
  Line 1-3/RConn3 -- Line 2-6/LConn3 -- BUS 5/LConn3 -- Line 5-1/LConn3 -- Line 4-1/LConn3
  BUS 7/LConn2 -- Line 4-2/LConn2 -- Line 7-1/RConn2 -- Line 7-2/RConn2
  Load Flow Bus32/LConn1 -- GEN 8/RConn1 -- BUS 8/RConn1
  Line 9-2/LConn1 -- BUS 14/LConn1 -- Line 13-1/RConn1
  Line 2-2/RConn2 -- Line 3-1/RConn2 -- Line 4-1/RConn2 -- BUS 4/LConn2 -- Line 4-3/RConn2 -- Line 4-2/RConn2
  Line 1-3/RConn2 -- BUS 5/LConn2 -- Line 5-1/LConn2 -- Line 4-1/LConn2 -- Line 2-6/LConn2
  Line 2-2/RConn3 -- Line 4-1/RConn3 -- Line 3-1/RConn3 -- BUS 4/LConn3 -- Line 4-3/RConn3 -- Line 4-2/RConn3
  Line 9-1/LConn3 -- BUS 10/LConn3 -- Line 10-1/LConn3
  Line 2-2/LConn2 -- BUS 2/RConn2 -- Line 2-1/LConn2 -- Line 1-1/RConn2 -- Line 2-6/RConn2
  Line 10-1/RConn1 -- Line 6-1/LConn1 -- BUS 11/LConn1
  Load Flow Bus31/LConn1 -- LOAD 10/LConn1 -- BUS 10/RConn1
  Load Flow Bus33/LConn1 -- " 1"/LConn1 -- LOAD 9/LConn1 -- BUS 9/RConn1
  Line 1-1/LConn1 -- BUS 1/RConn1 -- Line 1-3/LConn1
  BUS 6/LConn1 -- Line 6-1/RConn1 -- Line 5-1/RConn1 -- Line 6-3/RConn1 -- Line 6-2/RConn1
  BUS 3/LConn2 -- LOAD 3/LConn2 -- GEN 3/RConn2
  Line 2-2/LConn3 -- BUS 2/RConn3 -- Line 2-1/LConn3 -- Line 1-1/RConn3 -- Line 2-6/RConn3
  BUS 2/LConn2 -- LOAD 2/LConn2 -- GEN 2/RConn2
  Line 1-1/LConn3 -- BUS 1/RConn3 -- Line 1-3/LConn3
  BUS 3/LConn1 -- Load Flow Bus27/LConn1 -- LOAD 3/LConn1 -- GEN 3/RConn1
  GEN 6/RConn3 -- LOAD 6/LConn3 -- BUS 6/RConn3
  GEN 6/RConn2 -- LOAD 6/LConn2 -- BUS 6/RConn2
  Line 12-1/LConn1 -- Line 6-3/LConn1 -- BUS 13/LConn1 -- Line 13-1/LConn1
  Line 9-1/LConn1 -- BUS 10/LConn1 -- Line 10-1/LConn1
  Load Flow Bus28/LConn1 -- LOAD 4/LConn1 -- BUS 4/RConn1
  LOAD 9/LConn3 -- " 1"/LConn3 -- BUS 9/RConn3
  BUS 1/LConn1 -- SWING 1/RConn1 -- Load Flow Bus20/LConn1
  Line 6-2/LConn1 -- BUS 12/LConn1 -- Line 12-1/RConn1
  Load Flow Bus22/LConn1 -- LOAD 12/LConn1 -- BUS 12/RConn1
  GEN 2/RConn1 -- LOAD 2/LConn1 -- Load Flow Bus26/LConn1 -- BUS 2/LConn1
  Load Flow Bus21/LConn1 -- LOAD 11/LConn1 -- BUS 11/RConn1
  Line 3-1/LConn2 -- Line 2-1/RConn2 -- BUS 3/RConn2
  BUS 3/RConn1 -- Line 2-1/RConn1 -- Line 3-1/LConn1
  Load Flow Bus23/LConn1 -- LOAD 13/LConn1 -- BUS 13/RConn1
  LOAD 5/LConn2 -- BUS 5/RConn2
  LOAD 5/LConn3 -- BUS 5/RConn3
  LOAD 10/LConn3 -- BUS 10/RConn3
  LOAD 10/LConn2 -- BUS 10/RConn2
  LOAD 11/LConn2 -- BUS 11/RConn2
  LOAD 11/LConn3 -- BUS 11/RConn3
  LOAD 13/LConn2 -- BUS 13/RConn2
  LOAD 14/LConn3 -- BUS 14/RConn3
  LOAD 14/LConn2 -- BUS 14/RConn2
  BUS 8/RConn2 -- GEN 8/RConn2
  SWING 1/RConn2 -- BUS 1/LConn2
  BUS 8/RConn3 -- GEN 8/RConn3
  LOAD 5/LConn1 -- BUS 5/RConn1
  Line 7-1/LConn2 -- BUS 8/LConn2
  SWING 1/RConn3 -- BUS 1/LConn3
  LOAD 12/LConn2 -- BUS 12/RConn2
  Line 7-1/LConn1 -- BUS 8/LConn1
  LOAD 4/LConn2 -- BUS 4/RConn2
  Line 7-1/LConn3 -- BUS 8/LConn3
  LOAD 12/LConn3 -- BUS 12/RConn3
  LOAD 13/LConn3 -- BUS 13/RConn3
  LOAD 4/LConn3 -- BUS 4/RConn3
